simulink library "friction_resistance"  (R2020b)
settings: Solver=VariableStepAuto  StartTime=0.0  StopTime=10.0  RelTol=1e-3
values from neighbouring files (symbols this model uses):
  fr = 0.015    [Projektskript.m]    (also in init.m)
  g = 9.81    [Projektskript.m]    (also in init.m)
  m = 2000    [Projektskript.m]    (also in init.m)
settings Model: Creator=janbantle  LastModifiedBy=Johnathy

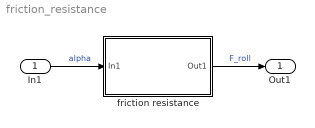
== system friction_resistance ==
  In1 : Inport
  "friction resistance " : Subsystem
  Out1 : Outport
  wires:
  In1/1 -> "friction resistance "/1(In1)  "alpha"
  "friction resistance "/1(Out1) -> Out1/1  "F_roll"

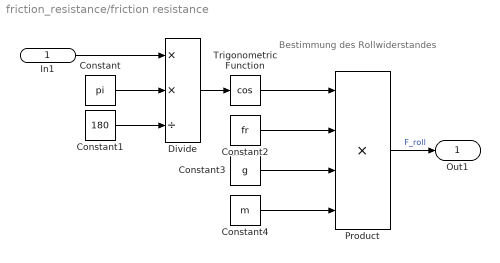
== system friction_resistance/friction resistance  ==
  note: Bestimmung des Rollwiderstandes
  In1 : Inport
  Constant : Constant  Value=pi
  Constant1 : Constant  Value=180
  Constant2 : Constant  Value=fr
  Constant3 : Constant  Value=g
  Constant4 : Constant  Value=m
  Divide : Product  Inputs=**/
  Product : Product  Inputs=4
  Trigonometric Function : Trigonometry  Operator=cos
  Out1 : Outport
  wires:
  Divide/1 -> Trigonometric Function/1
  In1/1 -> Divide/1
  Constant/1 -> Divide/2
  Product/1 -> Out1/1  "F_roll"
  Constant4/1 -> Product/4
  Constant3/1 -> Product/3
  Constant2/1 -> Product/2
  Constant1/1 -> Divide/3
  Trigonometric Function/1 -> Product/1
